simulink library "scp"  (R2021b)
settings: Solver=VariableStepAuto  StartTime=0.0  StopTime=10.0  RelTol=1e-3
libraries: FVT_lib x4
settings Model: Creator=FVT23118  LastModifiedBy=FVT23118

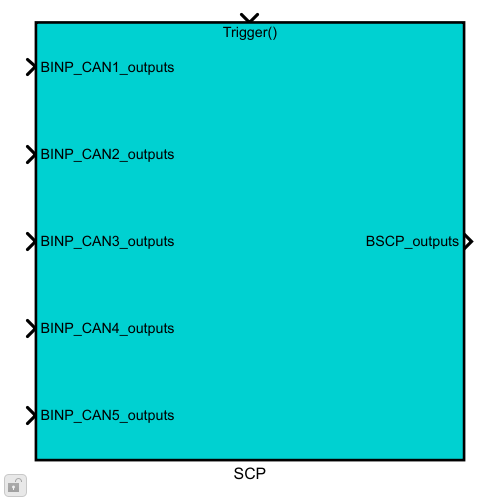
[thumbnail: Simulink's stored preview of the top-level diagram]
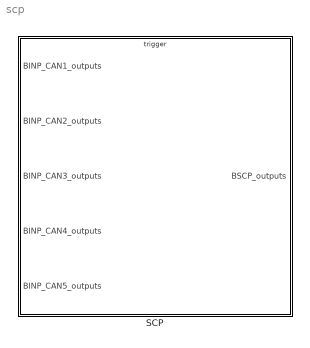
== system scp ==
  SCP : Subsystem

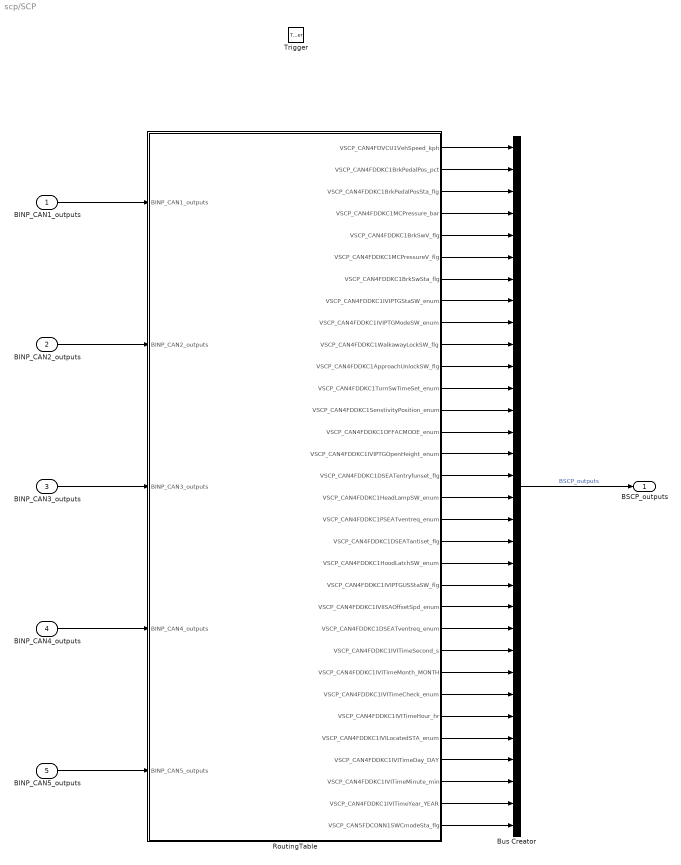
== system scp/SCP ==
  BINP_CAN1_outputs : Inport  OutDataTypeStr=Bus: BINP_CAN1_outputs
  BINP_CAN2_outputs : Inport  Port=2  OutDataTypeStr=Bus: BINP_CAN2_outputs
  BINP_CAN3_outputs : Inport  Port=3  OutDataTypeStr=Bus: BINP_CAN3_outputs
  BINP_CAN4_outputs : Inport  Port=4  OutDataTypeStr=Bus: BINP_CAN4_outputs
  BINP_CAN5_outputs : Inport  Port=5  OutDataTypeStr=Bus: BINP_CAN5_outputs
  Trigger : TriggerPort  TriggerType=function-call  VariantControl=(inherit)  PortDimensions=1
  Bus Creator : BusCreator  Inputs=32
  RoutingTable : Subsystem
  BSCP_outputs : Outport  OutDataTypeStr=Bus: BSCP_outputs
  wires:
  BINP_CAN4_outputs/1 -> RoutingTable/4(BINP_CAN4_outputs)
  BINP_CAN3_outputs/1 -> RoutingTable/3(BINP_CAN3_outputs)
  BINP_CAN1_outputs/1 -> RoutingTable/1(BINP_CAN1_outputs)
  BINP_CAN5_outputs/1 -> RoutingTable/5(BINP_CAN5_outputs)
  Bus Creator/1 -> BSCP_outputs/1  "BSCP_outputs"
  RoutingTable/30(VSCP_CAN4FDDKC1IVITimeMinute_min) -> Bus Creator/30
  RoutingTable/29(VSCP_CAN4FDDKC1IVITimeDay_DAY) -> Bus Creator/29
  RoutingTable/25(VSCP_CAN4FDDKC1IVITimeMonth_MONTH) -> Bus Creator/25
  RoutingTable/24(VSCP_CAN4FDDKC1IVITimeSecond_s) -> Bus Creator/24
  RoutingTable/23(VSCP_CAN4FDDKC1DSEATventreq_enum) -> Bus Creator/23
  RoutingTable/18(VSCP_CAN4FDDKC1PSEATventreq_enum) -> Bus Creator/18
  RoutingTable/20(VSCP_CAN4FDDKC1HoodLatchSW_enum) -> Bus Creator/20
  RoutingTable/19(VSCP_CAN4FDDKC1DSEATantiset_flg) -> Bus Creator/19
  RoutingTable/26(VSCP_CAN4FDDKC1IVITimeCheck_enum) -> Bus Creator/26
  RoutingTable/22(VSCP_CAN4FDDKC1IVIISAOffsetSpd_enum) -> Bus Creator/22
  RoutingTable/16(VSCP_CAN4FDDKC1DSEATentryfunset_flg) -> Bus Creator/16
  RoutingTable/17(VSCP_CAN4FDDKC1HeadLampSW_enum) -> Bus Creator/17
  RoutingTable/14(VSCP_CAN4FDDKC1OFFACMODE_enum) -> Bus Creator/14
  RoutingTable/13(VSCP_CAN4FDDKC1SenstivityPosition_enum) -> Bus Creator/13
  RoutingTable/28(VSCP_CAN4FDDKC1IVILocatedSTA_enum) -> Bus Creator/28
  RoutingTable/15(VSCP_CAN4FDDKC1IVIPTGOpenHeight_enum) -> Bus Creator/15
  RoutingTable/21(VSCP_CAN4FDDKC1IVIPTGUSStaSW_flg) -> Bus Creator/21
  RoutingTable/5(VSCP_CAN4FDDKC1BrkSwV_flg) -> Bus Creator/5
  RoutingTable/31(VSCP_CAN4FDDKC1IVITimeYear_YEAR) -> Bus Creator/31
  RoutingTable/10(VSCP_CAN4FDDKC1WalkawayLockSW_flg) -> Bus Creator/10
  RoutingTable/12(VSCP_CAN4FDDKC1TurnSwTimeSet_enum) -> Bus Creator/12
  RoutingTable/11(VSCP_CAN4FDDKC1ApproachUnlockSW_flg) -> Bus Creator/11
  RoutingTable/9(VSCP_CAN4FDDKC1IVIPTGModeSW_enum) -> Bus Creator/9
  RoutingTable/7(VSCP_CAN4FDDKC1BrkSwSta_flg) -> Bus Creator/7
  RoutingTable/4(VSCP_CAN4FDDKC1MCPressure_bar) -> Bus Creator/4
  RoutingTable/8(VSCP_CAN4FDDKC1IVIPTGStaSW_enum) -> Bus Creator/8
  RoutingTable/1(VSCP_CAN4FDVCU1VehSpeed_kph) -> Bus Creator/1
  RoutingTable/27(VSCP_CAN4FDDKC1IVITimeHour_hr) -> Bus Creator/27
  RoutingTable/6(VSCP_CAN4FDDKC1MCPressureV_flg) -> Bus Creator/6
  BINP_CAN2_outputs/1 -> RoutingTable/2(BINP_CAN2_outputs)
  RoutingTable/3(VSCP_CAN4FDDKC1BrkPedalPosSta_flg) -> Bus Creator/3
  RoutingTable/2(VSCP_CAN4FDDKC1BrkPedalPos_pct) -> Bus Creator/2
  RoutingTable/32(VSCP_CAN5FDCONN1SWCmodeSta_flg) -> Bus Creator/32

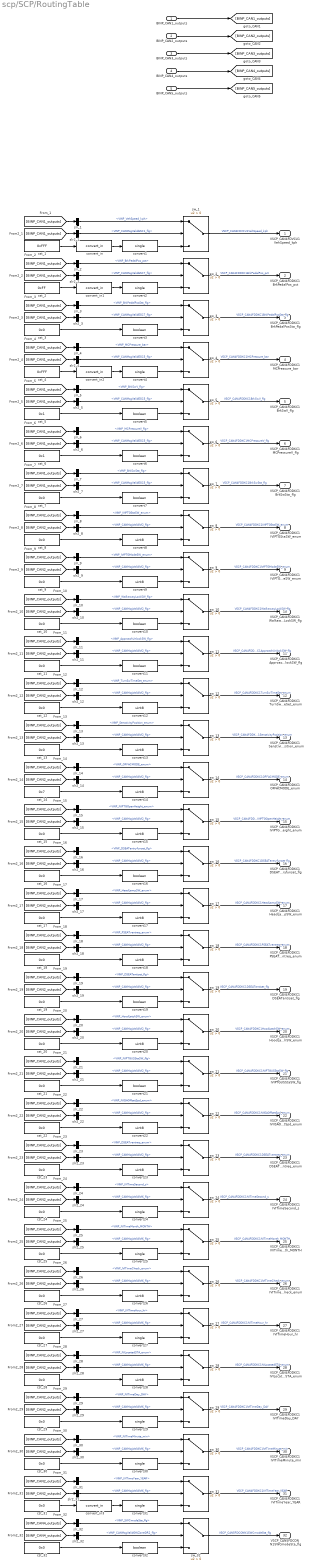
== system scp/SCP/RoutingTable ==
  BINP_CAN1_outputs : Inport
  BINP_CAN2_outputs : Inport  Port=2
  BINP_CAN3_outputs : Inport  Port=3
  BINP_CAN4_outputs : Inport  Port=4
  BINP_CAN5_outputs : Inport  Port=5
  convert{1..2,4,24..25,27,29..31} (9 alike) : DataTypeConversion  OutDataTypeStr=single
  convert{3,5..7,10..11,16,19,21,32} (10 alike) : DataTypeConversion  OutDataTypeStr=boolean
  convert{8..9,12..15,17..18,20,22..23,26,28} (13 alike) : DataTypeConversion  OutDataTypeStr=uint8
  convert_in : FVT_lib/hal/convert_in  gain=0.125  offset=0
  convert_in1 : FVT_lib/hal/convert_in  gain=0.4  offset=0
  convert_in2 : FVT_lib/hal/convert_in  gain=0.1  offset=-9.7
  convert_in3 : FVT_lib/hal/convert_in  gain=1  offset=2000
  cst_1 : Constant  Value=0xFFF
  cst_{3,7..13,15..32} (26 alike) : Constant  Value=0x0
  cst_14 : Constant  Value=0x7
  cst_2 : Constant  Value=0xFF
  cst_4 : Constant  Value=0xFFF
  cst_5 : Constant  Value=0x1
  cst_6 : Constant  Value=0x1
  slr2_1 : BusSelector  OutputSignals=VINP_CANMsgValidESC1_flg
  slr2_{8..23} (16 alike) : BusSelector  OutputSignals=VINP_CANMsgValidIVI2_flg
  slr2_2 : BusSelector  OutputSignals=VINP_CANMsgValidESC7_flg
  slr2_{24..31} (8 alike) : BusSelector  OutputSignals=VINP_CANMsgValidIVI6_flg
  slr2_3 : BusSelector  OutputSignals=VINP_CANMsgValidESC7_flg
  slr2_32 : BusSelector  OutputSignals=VINP_CANMsgValidGWZoneDR2_flg
  slr2_{4..7} (4 alike) : BusSelector  OutputSignals=VINP_CANMsgValidESC5_flg
  slr_1 : BusSelector  OutputSignals=VINP_VehSpeed_kph
  slr_10 : BusSelector  OutputSignals=VINP_WalkawayLockSW_flg
  slr_11 : BusSelector  OutputSignals=VINP_ApproachUnlockSW_flg
  slr_12 : BusSelector  OutputSignals=VINP_TurnSwTimeSet_enum
  slr_13 : BusSelector  OutputSignals=VINP_SenstivityPosition_enum
  slr_14 : BusSelector  OutputSignals=VINP_OFFACMODE_enum
  slr_15 : BusSelector  OutputSignals=VINP_IVIPTGOpenHeight_enum
  slr_16 : BusSelector  OutputSignals=VINP_DSEATentryfunset_flg
  slr_17 : BusSelector  OutputSignals=VINP_HeadLampSW_enum
  slr_18 : BusSelector  OutputSignals=VINP_PSEATventreq_enum
  slr_19 : BusSelector  OutputSignals=VINP_DSEATantiset_flg
  slr_2 : BusSelector  OutputSignals=VINP_BrkPedalPos_pct
  slr_20 : BusSelector  OutputSignals=VINP_HoodLatchSW_enum
  slr_21 : BusSelector  OutputSignals=VINP_IVIPTGUSStaSW_flg
  slr_22 : BusSelector  OutputSignals=VINP_IVIISAOffsetSpd_enum
  slr_23 : BusSelector  OutputSignals=VINP_DSEATventreq_enum
  slr_24 : BusSelector  OutputSignals=VINP_IVITimeSecond_s
  slr_25 : BusSelector  OutputSignals=VINP_IVITimeMonth_MONTH
  slr_26 : BusSelector  OutputSignals=VINP_IVITimeCheck_enum
  slr_27 : BusSelector  OutputSignals=VINP_IVITimeHour_hr
  slr_28 : BusSelector  OutputSignals=VINP_IVILocatedSTA_enum
  slr_29 : BusSelector  OutputSignals=VINP_IVITimeDay_DAY
  slr_3 : BusSelector  OutputSignals=VINP_BrkPedalPosSta_flg
  slr_30 : BusSelector  OutputSignals=VINP_IVITimeMinute_min
  slr_31 : BusSelector  OutputSignals=VINP_IVITimeYear_YEAR
  slr_32 : BusSelector  OutputSignals=VINP_SWCmodeSta_flg
  slr_4 : BusSelector  OutputSignals=VINP_MCPressure_bar
  slr_5 : BusSelector  OutputSignals=VINP_BrkSwV_flg
  slr_6 : BusSelector  OutputSignals=VINP_MCPressureV_flg
  slr_7 : BusSelector  OutputSignals=VINP_BrkSwSta_flg
  slr_8 : BusSelector  OutputSignals=VINP_IVIPTGStaSW_enum
  slr_9 : BusSelector  OutputSignals=VINP_IVIPTGModeSW_enum
  sw_{1..32} (32 alike) : Switch  Criteria=u2 > Threshold
  VSCP_CAN4FDVCU1VehSpeed_kph : Outport
  VSCP_CAN4FDDKC1BrkPedalPos_pct : Outport  Port=2
  VSCP_CAN4FDDKC1BrkPedalPosSta_flg : Outport  Port=3
  VSCP_CAN4FDDKC1MCPressure_bar : Outport  Port=4
  VSCP_CAN4FDDKC1BrkSwV_flg : Outport  Port=5
  VSCP_CAN4FDDKC1MCPressureV_flg : Outport  Port=6
  VSCP_CAN4FDDKC1BrkSwSta_flg : Outport  Port=7
  VSCP_CAN4FDDKC1IVIPTGStaSW_enum : Outport  Port=8
  VSCP_CAN4FDDKC1IVIPTGModeSW_enum : Outport  Port=9
  VSCP_CAN4FDDKC1WalkawayLockSW_flg : Outport  Port=10
  VSCP_CAN4FDDKC1ApproachUnlockSW_flg : Outport  Port=11
  VSCP_CAN4FDDKC1TurnSwTimeSet_enum : Outport  Port=12
  VSCP_CAN4FDDKC1SenstivityPosition_enum : Outport  Port=13
  VSCP_CAN4FDDKC1OFFACMODE_enum : Outport  Port=14
  VSCP_CAN4FDDKC1IVIPTGOpenHeight_enum : Outport  Port=15
  VSCP_CAN4FDDKC1DSEATentryfunset_flg : Outport  Port=16
  VSCP_CAN4FDDKC1HeadLampSW_enum : Outport  Port=17
  VSCP_CAN4FDDKC1PSEATventreq_enum : Outport  Port=18
  VSCP_CAN4FDDKC1DSEATantiset_flg : Outport  Port=19
  VSCP_CAN4FDDKC1HoodLatchSW_enum : Outport  Port=20
  VSCP_CAN4FDDKC1IVIPTGUSStaSW_flg : Outport  Port=21
  VSCP_CAN4FDDKC1IVIISAOffsetSpd_enum : Outport  Port=22
  VSCP_CAN4FDDKC1DSEATventreq_enum : Outport  Port=23
  VSCP_CAN4FDDKC1IVITimeSecond_s : Outport  Port=24
  VSCP_CAN4FDDKC1IVITimeMonth_MONTH : Outport  Port=25
  VSCP_CAN4FDDKC1IVITimeCheck_enum : Outport  Port=26
  VSCP_CAN4FDDKC1IVITimeHour_hr : Outport  Port=27
  VSCP_CAN4FDDKC1IVILocatedSTA_enum : Outport  Port=28
  VSCP_CAN4FDDKC1IVITimeDay_DAY : Outport  Port=29
  VSCP_CAN4FDDKC1IVITimeMinute_min : Outport  Port=30
  VSCP_CAN4FDDKC1IVITimeYear_YEAR : Outport  Port=31
  VSCP_CAN5FDCONN1SWCmodeSta_flg : Outport  Port=32
  wires:
  BINP_CAN1_outputs/1 -> [BINP_CAN1_outputs]
  BINP_CAN2_outputs/1 -> [BINP_CAN2_outputs]
  BINP_CAN3_outputs/1 -> [BINP_CAN3_outputs]
  BINP_CAN4_outputs/1 -> [BINP_CAN4_outputs]
  BINP_CAN5_outputs/1 -> [BINP_CAN5_outputs]
  [BINP_CAN1_outputs] -> slr_1/1
  slr_1/1 -> sw_1/1  "<VINP_VehSpeed_kph>"
  [BINP_CAN1_outputs] -> slr2_1/1
  slr2_1/1 -> sw_1/2  "<VINP_CANMsgValidESC1_flg>"
  cst_1/1 -> convert_in/1
  convert_in/1 -> convert1/1
  convert1/1 -> sw_1/3
  sw_1/1 -> VSCP_CAN4FDVCU1VehSpeed_kph/1  "VSCP_CAN4FDVCU1VehSpeed_kph"
  [BINP_CAN1_outputs] -> slr_2/1
  slr_2/1 -> sw_2/1  "<VINP_BrkPedalPos_pct>"
  [BINP_CAN1_outputs] -> slr2_2/1
  slr2_2/1 -> sw_2/2  "<VINP_CANMsgValidESC7_flg>"
  cst_2/1 -> convert_in1/1
  convert_in1/1 -> convert2/1
  convert2/1 -> sw_2/3
  sw_2/1 -> VSCP_CAN4FDDKC1BrkPedalPos_pct/1  "VSCP_CAN4FDDKC1BrkPedalPos_pct"
  [BINP_CAN1_outputs] -> slr_3/1
  slr_3/1 -> sw_3/1  "<VINP_BrkPedalPosSta_flg>"
  [BINP_CAN1_outputs] -> slr2_3/1
  slr2_3/1 -> sw_3/2  "<VINP_CANMsgValidESC7_flg>"
  cst_3/1 -> convert3/1
  convert3/1 -> sw_3/3
  sw_3/1 -> VSCP_CAN4FDDKC1BrkPedalPosSta_flg/1  "VSCP_CAN4FDDKC1BrkPedalPosSta_flg"
  [BINP_CAN1_outputs] -> slr_4/1
  slr_4/1 -> sw_4/1  "<VINP_MCPressure_bar>"
  [BINP_CAN1_outputs] -> slr2_4/1
  slr2_4/1 -> sw_4/2  "<VINP_CANMsgValidESC5_flg>"
  cst_4/1 -> convert_in2/1
  convert_in2/1 -> convert4/1
  convert4/1 -> sw_4/3
  sw_4/1 -> VSCP_CAN4FDDKC1MCPressure_bar/1  "VSCP_CAN4FDDKC1MCPressure_bar"
  [BINP_CAN1_outputs] -> slr_5/1
  slr_5/1 -> sw_5/1  "<VINP_BrkSwV_flg>"
  [BINP_CAN1_outputs] -> slr2_5/1
  slr2_5/1 -> sw_5/2  "<VINP_CANMsgValidESC5_flg>"
  cst_5/1 -> convert5/1
  convert5/1 -> sw_5/3
  sw_5/1 -> VSCP_CAN4FDDKC1BrkSwV_flg/1  "VSCP_CAN4FDDKC1BrkSwV_flg"
  [BINP_CAN1_outputs] -> slr_6/1
  slr_6/1 -> sw_6/1  "<VINP_MCPressureV_flg>"
  [BINP_CAN1_outputs] -> slr2_6/1
  slr2_6/1 -> sw_6/2  "<VINP_CANMsgValidESC5_flg>"
  cst_6/1 -> convert6/1
  convert6/1 -> sw_6/3
  sw_6/1 -> VSCP_CAN4FDDKC1MCPressureV_flg/1  "VSCP_CAN4FDDKC1MCPressureV_flg"
  [BINP_CAN1_outputs] -> slr_7/1
  slr_7/1 -> sw_7/1  "<VINP_BrkSwSta_flg>"
  [BINP_CAN1_outputs] -> slr2_7/1
  slr2_7/1 -> sw_7/2  "<VINP_CANMsgValidESC5_flg>"
  cst_7/1 -> convert7/1
  convert7/1 -> sw_7/3
  sw_7/1 -> VSCP_CAN4FDDKC1BrkSwSta_flg/1  "VSCP_CAN4FDDKC1BrkSwSta_flg"
  [BINP_CAN2_outputs] -> slr_8/1
  slr_8/1 -> sw_8/1  "<VINP_IVIPTGStaSW_enum>"
  [BINP_CAN2_outputs] -> slr2_8/1
  slr2_8/1 -> sw_8/2  "<VINP_CANMsgValidIVI2_flg>"
  cst_8/1 -> convert8/1
  convert8/1 -> sw_8/3
  sw_8/1 -> VSCP_CAN4FDDKC1IVIPTGStaSW_enum/1  "VSCP_CAN4FDDKC1IVIPTGStaSW_enum"
  [BINP_CAN2_outputs] -> slr_9/1
  slr_9/1 -> sw_9/1  "<VINP_IVIPTGModeSW_enum>"
  [BINP_CAN2_outputs] -> slr2_9/1
  slr2_9/1 -> sw_9/2  "<VINP_CANMsgValidIVI2_flg>"
  cst_9/1 -> convert9/1
  convert9/1 -> sw_9/3
  sw_9/1 -> VSCP_CAN4FDDKC1IVIPTGModeSW_enum/1  "VSCP_CAN4FDDKC1IVIPTGModeSW_enum"
  [BINP_CAN2_outputs] -> slr_10/1
  slr_10/1 -> sw_10/1  "<VINP_WalkawayLockSW_flg>"
  [BINP_CAN2_outputs] -> slr2_10/1
  slr2_10/1 -> sw_10/2  "<VINP_CANMsgValidIVI2_flg>"
  cst_10/1 -> convert10/1
  convert10/1 -> sw_10/3
  sw_10/1 -> VSCP_CAN4FDDKC1WalkawayLockSW_flg/1  "VSCP_CAN4FDDKC1WalkawayLockSW_flg"
  [BINP_CAN2_outputs] -> slr_11/1
  slr_11/1 -> sw_11/1  "<VINP_ApproachUnlockSW_flg>"
  [BINP_CAN2_outputs] -> slr2_11/1
  slr2_11/1 -> sw_11/2  "<VINP_CANMsgValidIVI2_flg>"
  cst_11/1 -> convert11/1
  convert11/1 -> sw_11/3
  sw_11/1 -> VSCP_CAN4FDDKC1ApproachUnlockSW_flg/1  "VSCP_CAN4FDDKC1ApproachUnlockSW_flg"
  [BINP_CAN2_outputs] -> slr_12/1
  slr_12/1 -> sw_12/1  "<VINP_TurnSwTimeSet_enum>"
  [BINP_CAN2_outputs] -> slr2_12/1
  slr2_12/1 -> sw_12/2  "<VINP_CANMsgValidIVI2_flg>"
  cst_12/1 -> convert12/1
  convert12/1 -> sw_12/3
  sw_12/1 -> VSCP_CAN4FDDKC1TurnSwTimeSet_enum/1  "VSCP_CAN4FDDKC1TurnSwTimeSet_enum"
  [BINP_CAN2_outputs] -> slr_13/1
  slr_13/1 -> sw_13/1  "<VINP_SenstivityPosition_enum>"
  [BINP_CAN2_outputs] -> slr2_13/1
  slr2_13/1 -> sw_13/2  "<VINP_CANMsgValidIVI2_flg>"
  cst_13/1 -> convert13/1
  convert13/1 -> sw_13/3
  sw_13/1 -> VSCP_CAN4FDDKC1SenstivityPosition_enum/1  "VSCP_CAN4FDDKC1SenstivityPosition_enum"
  [BINP_CAN2_outputs] -> slr_14/1
  slr_14/1 -> sw_14/1  "<VINP_OFFACMODE_enum>"
  [BINP_CAN2_outputs] -> slr2_14/1
  slr2_14/1 -> sw_14/2  "<VINP_CANMsgValidIVI2_flg>"
  cst_14/1 -> convert14/1
  convert14/1 -> sw_14/3
  sw_14/1 -> VSCP_CAN4FDDKC1OFFACMODE_enum/1  "VSCP_CAN4FDDKC1OFFACMODE_enum"
  [BINP_CAN2_outputs] -> slr_15/1
  slr_15/1 -> sw_15/1  "<VINP_IVIPTGOpenHeight_enum>"
  [BINP_CAN2_outputs] -> slr2_15/1
  slr2_15/1 -> sw_15/2  "<VINP_CANMsgValidIVI2_flg>"
  cst_15/1 -> convert15/1
  convert15/1 -> sw_15/3
  sw_15/1 -> VSCP_CAN4FDDKC1IVIPTGOpenHeight_enum/1  "VSCP_CAN4FDDKC1IVIPTGOpenHeight_enum"
  [BINP_CAN2_outputs] -> slr_16/1
  slr_16/1 -> sw_16/1  "<VINP_DSEATentryfunset_flg>"
  [BINP_CAN2_outputs] -> slr2_16/1
  slr2_16/1 -> sw_16/2  "<VINP_CANMsgValidIVI2_flg>"
  cst_16/1 -> convert16/1
  convert16/1 -> sw_16/3
  sw_16/1 -> VSCP_CAN4FDDKC1DSEATentryfunset_flg/1  "VSCP_CAN4FDDKC1DSEATentryfunset_flg"
  [BINP_CAN2_outputs] -> slr_17/1
  slr_17/1 -> sw_17/1  "<VINP_HeadLampSW_enum>"
  [BINP_CAN2_outputs] -> slr2_17/1
  slr2_17/1 -> sw_17/2  "<VINP_CANMsgValidIVI2_flg>"
  cst_17/1 -> convert17/1
  convert17/1 -> sw_17/3
  sw_17/1 -> VSCP_CAN4FDDKC1HeadLampSW_enum/1  "VSCP_CAN4FDDKC1HeadLampSW_enum"
  [BINP_CAN2_outputs] -> slr_18/1
  slr_18/1 -> sw_18/1  "<VINP_PSEATventreq_enum>"
  [BINP_CAN2_outputs] -> slr2_18/1
  slr2_18/1 -> sw_18/2  "<VINP_CANMsgValidIVI2_flg>"
  cst_18/1 -> convert18/1
  convert18/1 -> sw_18/3
  sw_18/1 -> VSCP_CAN4FDDKC1PSEATventreq_enum/1  "VSCP_CAN4FDDKC1PSEATventreq_enum"
  [BINP_CAN2_outputs] -> slr_19/1
  slr_19/1 -> sw_19/1  "<VINP_DSEATantiset_flg>"
  [BINP_CAN2_outputs] -> slr2_19/1
  slr2_19/1 -> sw_19/2  "<VINP_CANMsgValidIVI2_flg>"
  cst_19/1 -> convert19/1
  convert19/1 -> sw_19/3
  sw_19/1 -> VSCP_CAN4FDDKC1DSEATantiset_flg/1  "VSCP_CAN4FDDKC1DSEATantiset_flg"
  [BINP_CAN2_outputs] -> slr_20/1
  slr_20/1 -> sw_20/1  "<VINP_HoodLatchSW_enum>"
  [BINP_CAN2_outputs] -> slr2_20/1
  slr2_20/1 -> sw_20/2  "<VINP_CANMsgValidIVI2_flg>"
  cst_20/1 -> convert20/1
  convert20/1 -> sw_20/3
  sw_20/1 -> VSCP_CAN4FDDKC1HoodLatchSW_enum/1  "VSCP_CAN4FDDKC1HoodLatchSW_enum"
  [BINP_CAN2_outputs] -> slr_21/1
  slr_21/1 -> sw_21/1  "<VINP_IVIPTGUSStaSW_flg>"
  [BINP_CAN2_outputs] -> slr2_21/1
  slr2_21/1 -> sw_21/2  "<VINP_CANMsgValidIVI2_flg>"
  cst_21/1 -> convert21/1
  convert21/1 -> sw_21/3
  sw_21/1 -> VSCP_CAN4FDDKC1IVIPTGUSStaSW_flg/1  "VSCP_CAN4FDDKC1IVIPTGUSStaSW_flg"
  [BINP_CAN2_outputs] -> slr_22/1
  slr_22/1 -> sw_22/1  "<VINP_IVIISAOffsetSpd_enum>"
  [BINP_CAN2_outputs] -> slr2_22/1
  slr2_22/1 -> sw_22/2  "<VINP_CANMsgValidIVI2_flg>"
  cst_22/1 -> convert22/1
  convert22/1 -> sw_22/3
  sw_22/1 -> VSCP_CAN4FDDKC1IVIISAOffsetSpd_enum/1  "VSCP_CAN4FDDKC1IVIISAOffsetSpd_enum"
  [BINP_CAN2_outputs] -> slr_23/1
  slr_23/1 -> sw_23/1  "<VINP_DSEATventreq_enum>"
  [BINP_CAN2_outputs] -> slr2_23/1
  slr2_23/1 -> sw_23/2  "<VINP_CANMsgValidIVI2_flg>"
  cst_23/1 -> convert23/1
  convert23/1 -> sw_23/3
  sw_23/1 -> VSCP_CAN4FDDKC1DSEATventreq_enum/1  "VSCP_CAN4FDDKC1DSEATventreq_enum"
  [BINP_CAN2_outputs] -> slr_24/1
  slr_24/1 -> sw_24/1  "<VINP_IVITimeSecond_s>"
  [BINP_CAN2_outputs] -> slr2_24/1
  slr2_24/1 -> sw_24/2  "<VINP_CANMsgValidIVI6_flg>"
  cst_24/1 -> convert24/1
  convert24/1 -> sw_24/3
  sw_24/1 -> VSCP_CAN4FDDKC1IVITimeSecond_s/1  "VSCP_CAN4FDDKC1IVITimeSecond_s"
  [BINP_CAN2_outputs] -> slr_25/1
  slr_25/1 -> sw_25/1  "<VINP_IVITimeMonth_MONTH>"
  [BINP_CAN2_outputs] -> slr2_25/1
  slr2_25/1 -> sw_25/2  "<VINP_CANMsgValidIVI6_flg>"
  cst_25/1 -> convert25/1
  convert25/1 -> sw_25/3
  sw_25/1 -> VSCP_CAN4FDDKC1IVITimeMonth_MONTH/1  "VSCP_CAN4FDDKC1IVITimeMonth_MONTH"
  [BINP_CAN2_outputs] -> slr_26/1
  slr_26/1 -> sw_26/1  "<VINP_IVITimeCheck_enum>"
  [BINP_CAN2_outputs] -> slr2_26/1
  slr2_26/1 -> sw_26/2  "<VINP_CANMsgValidIVI6_flg>"
  cst_26/1 -> convert26/1
  convert26/1 -> sw_26/3
  sw_26/1 -> VSCP_CAN4FDDKC1IVITimeCheck_enum/1  "VSCP_CAN4FDDKC1IVITimeCheck_enum"
  [BINP_CAN2_outputs] -> slr_27/1
  slr_27/1 -> sw_27/1  "<VINP_IVITimeHour_hr>"
  [BINP_CAN2_outputs] -> slr2_27/1
  slr2_27/1 -> sw_27/2  "<VINP_CANMsgValidIVI6_flg>"
  cst_27/1 -> convert27/1
  convert27/1 -> sw_27/3
  sw_27/1 -> VSCP_CAN4FDDKC1IVITimeHour_hr/1  "VSCP_CAN4FDDKC1IVITimeHour_hr"
  [BINP_CAN2_outputs] -> slr_28/1
  slr_28/1 -> sw_28/1  "<VINP_IVILocatedSTA_enum>"
  [BINP_CAN2_outputs] -> slr2_28/1
  slr2_28/1 -> sw_28/2  "<VINP_CANMsgValidIVI6_flg>"
  cst_28/1 -> convert28/1
  convert28/1 -> sw_28/3
  sw_28/1 -> VSCP_CAN4FDDKC1IVILocatedSTA_enum/1  "VSCP_CAN4FDDKC1IVILocatedSTA_enum"
  [BINP_CAN2_outputs] -> slr_29/1
  slr_29/1 -> sw_29/1  "<VINP_IVITimeDay_DAY>"
  [BINP_CAN2_outputs] -> slr2_29/1
  slr2_29/1 -> sw_29/2  "<VINP_CANMsgValidIVI6_flg>"
  cst_29/1 -> convert29/1
  convert29/1 -> sw_29/3
  sw_29/1 -> VSCP_CAN4FDDKC1IVITimeDay_DAY/1  "VSCP_CAN4FDDKC1IVITimeDay_DAY"
  [BINP_CAN2_outputs] -> slr_30/1
  slr_30/1 -> sw_30/1  "<VINP_IVITimeMinute_min>"
  [BINP_CAN2_outputs] -> slr2_30/1
  slr2_30/1 -> sw_30/2  "<VINP_CANMsgValidIVI6_flg>"
  cst_30/1 -> convert30/1
  convert30/1 -> sw_30/3
  sw_30/1 -> VSCP_CAN4FDDKC1IVITimeMinute_min/1  "VSCP_CAN4FDDKC1IVITimeMinute_min"
  [BINP_CAN2_outputs] -> slr_31/1
  slr_31/1 -> sw_31/1  "<VINP_IVITimeYear_YEAR>"
  [BINP_CAN2_outputs] -> slr2_31/1
  slr2_31/1 -> sw_31/2  "<VINP_CANMsgValidIVI6_flg>"
  cst_31/1 -> convert_in3/1
  convert_in3/1 -> convert31/1
  convert31/1 -> sw_31/3
  sw_31/1 -> VSCP_CAN4FDDKC1IVITimeYear_YEAR/1  "VSCP_CAN4FDDKC1IVITimeYear_YEAR"
  [BINP_CAN4_outputs] -> slr_32/1
  slr_32/1 -> sw_32/1  "<VINP_SWCmodeSta_flg>"
  [BINP_CAN4_outputs] -> slr2_32/1
  slr2_32/1 -> sw_32/2  "<VINP_CANMsgValidGWZoneDR2_flg>"
  cst_32/1 -> convert32/1
  convert32/1 -> sw_32/3
  sw_32/1 -> VSCP_CAN5FDCONN1SWCmodeSta_flg/1  "VSCP_CAN5FDCONN1SWCmodeSta_flg"
